simulink model "EHB_MOTOR"  (R2023b)
settings: Solver=FixedStepDiscrete  StartTime=0.0  StopTime=inf  FixedStep=0.0001  RelTol=1e-3  EnableMultiTasking=on
undefined symbols (not defined in the file): CAN_EHB_VCU0x125, CAN_EHB_VCU0x126, CAN_id0x120_Data, Cos_Table, Cos_Table1, EHB_DTC_status, R, Sin_BreakPoint, Sin_BreakPoint1, Sin_Table, Sin_Table1, T
libraries: simulink x30
(part 5 of 9)

== system EHB_MOTOR/EHB_MOTOR_PRO/DIAG/EHBDiag/Subsystem ==
  note: 电源电压过高
  note: 11V
  note: 16V
  note: 电源电压过低
  note: 9V
  note: 14V
  In1 : Inport
  function : TriggerPort  TriggerType=function-call  VariantControl=Variant
  Constant{,1..3} (4 alike) : Constant  Value=0  OutDataTypeStr=uint8
  Data Store Memory1 : DataStoreMemory  DataStoreName=EHBVoltage_C  ReadBeforeWriteMsg=warning  WriteAfterWriteMsg=warning  WriteAfterReadMsg=warning  ShowAdditionalParam=off  OutDataTypeStr=uint16
  Data Store Memory2 : DataStoreMemory  DataStoreName=EHBVoltageMIN2_C  ReadBeforeWriteMsg=warning  WriteAfterWriteMsg=warning  WriteAfterReadMsg=warning  ShowAdditionalParam=off  OutDataTypeStr=uint16
  Data Store Memory3 : DataStoreMemory  DataStoreName=EHBVoltageMAX2_C  ReadBeforeWriteMsg=warning  WriteAfterWriteMsg=warning  WriteAfterReadMsg=warning  ShowAdditionalParam=off  OutDataTypeStr=uint16
  Data Store Memory4 : DataStoreMemory  DataStoreName=EHBVoltageMIN1_C  ReadBeforeWriteMsg=warning  WriteAfterWriteMsg=warning  WriteAfterReadMsg=warning  ShowAdditionalParam=off  OutDataTypeStr=uint16
  Data Store Memory5 : DataStoreMemory  DataStoreName=EHBVoltageMAX1_C  ReadBeforeWriteMsg=warning  WriteAfterWriteMsg=warning  WriteAfterReadMsg=warning  ShowAdditionalParam=off  OutDataTypeStr=uint16
  Data Store Read : DataStoreRead  DataStoreName=EHBVoltage_C  DataStoreElements=EHBVoltage_C  IndexOptions=Index vector (dialog)  Indices=1  OutputSizes=1
  Data Store Read1 : DataStoreRead  DataStoreName=EHBVoltageMIN1_C  DataStoreElements=EHBVoltageMIN1_C  IndexOptions=Index vector (dialog)  Indices=1  OutputSizes=1
  Data Store Read2 : DataStoreRead  DataStoreName=EHBVoltageMAX1_C  DataStoreElements=EHBVoltageMAX1_C  IndexOptions=Index vector (dialog)  Indices=1  OutputSizes=1
  Data Store Read3 : DataStoreRead  DataStoreName=EHBVoltageMAX2_C  DataStoreElements=EHBVoltageMAX2_C  IndexOptions=Index vector (dialog)  Indices=1  OutputSizes=1
  Data Store Read5 : DataStoreRead  DataStoreName=EHBVoltageMIN2_C  DataStoreElements=EHBVoltageMIN2_C  IndexOptions=Index vector (dialog)  Indices=1  OutputSizes=1
  ErrorSignalCount : Stateflow chart  TreatAsAtomicUnit=on
  ErrorSignalCount1 : Stateflow chart  TreatAsAtomicUnit=on
  ErrorSignalCount2 : Stateflow chart  TreatAsAtomicUnit=on
  ErrorSignalCount3 : Stateflow chart  TreatAsAtomicUnit=on
  Relational Operator : RelationalOperator  Operator=<  OutDataTypeStr=boolean  RndMeth=Simplest  InputSameDT=off
  Relational Operator1 : RelationalOperator  Operator=>  OutDataTypeStr=boolean  RndMeth=Simplest  InputSameDT=off
  Relational Operator2 : RelationalOperator  Operator=<  OutDataTypeStr=boolean  RndMeth=Simplest  InputSameDT=off
  Relational Operator3 : RelationalOperator  Operator=>  OutDataTypeStr=boolean  RndMeth=Simplest  InputSameDT=off
  EHBVoltageLow1 : Outport  VectorParamsAs1DForOutWhenUnconnected=off
  EHBVoltageLow2 : Outport  Port=2  VectorParamsAs1DForOutWhenUnconnected=off
  EHBVoltageHigh1 : Outport  Port=3  VectorParamsAs1DForOutWhenUnconnected=off
  EHBVoltageHigh2 : Outport  Port=4  VectorParamsAs1DForOutWhenUnconnected=off
  wires:
  Data Store Read1/1 -> Relational Operator/2
  In1/1 -> Relational Operator/1, Relational Operator2/1, Relational Operator1/1, Relational Operator3/1
  Data Store Read2/1 -> Relational Operator1/2
  ErrorSignalCount1/1(EHBVoltageMIN) -> EHBVoltageLow1/1
  Relational Operator/1 -> ErrorSignalCount1/1(EHBVoltage)
  Constant/1 -> ErrorSignalCount1/3(Recover)
  Constant1/1 -> ErrorSignalCount/3(Recover)
  Relational Operator1/1 -> ErrorSignalCount/1(EHBVoltage)
  ErrorSignalCount/1(EHBVoltageMAX) -> EHBVoltageHigh1/1
  Constant2/1 -> ErrorSignalCount2/3(Recover)
  Relational Operator2/1 -> ErrorSignalCount2/1(EHBVoltage)
  Data Store Read5/1 -> Relational Operator2/2
  Data Store Read/1 -> ErrorSignalCount1/2(EHBVoltageMIN_C), ErrorSignalCount2/2(EHBVoltageMIN_C), ErrorSignalCount3/2(EHBVoltageMAX_C), ErrorSignalCount/2(EHBVoltageMAX_C)
  Constant3/1 -> ErrorSignalCount3/3(Recover)
  Data Store Read3/1 -> Relational Operator3/2
  Relational Operator3/1 -> ErrorSignalCount3/1(EHBVoltage)
  ErrorSignalCount2/1(EHBVoltageMIN) -> EHBVoltageLow2/1
  ErrorSignalCount3/1(EHBVoltageMAX) -> EHBVoltageHigh2/1

== system EHB_MOTOR/EHB_MOTOR_PRO/DIAG/KL15VoltageDiag/Subsystem ==
  note: 电源电压过低
  note: 16V
  note: 10V
  note: 电源电压过高
  KL15Voltage : Inport
  function : TriggerPort  TriggerType=function-call  VariantControl=Variant
  Constant : Constant  Value=0  OutDataTypeStr=uint8
  Constant1 : Constant  Value=0  OutDataTypeStr=uint8
  Data Store Memory1 : DataStoreMemory  DataStoreName=KL15Voltage_C  ReadBeforeWriteMsg=warning  WriteAfterWriteMsg=warning  WriteAfterReadMsg=warning  ShowAdditionalParam=off  OutDataTypeStr=uint16
  Data Store Memory4 : DataStoreMemory  DataStoreName=KL15VoltageMIN_C  ReadBeforeWriteMsg=warning  WriteAfterWriteMsg=warning  WriteAfterReadMsg=warning  ShowAdditionalParam=off  OutDataTypeStr=uint16
  Data Store Memory5 : DataStoreMemory  DataStoreName=KL15VoltageMAX_C  ReadBeforeWriteMsg=warning  WriteAfterWriteMsg=warning  WriteAfterReadMsg=warning  ShowAdditionalParam=off  OutDataTypeStr=uint16
  Data Store Read : DataStoreRead  DataStoreName=KL15Voltage_C  DataStoreElements=KL15Voltage_C  IndexOptions=Index vector (dialog)  Indices=1  OutputSizes=1
  Data Store Read1 : DataStoreRead  DataStoreName=KL15VoltageMIN_C  DataStoreElements=KL15VoltageMIN_C  IndexOptions=Index vector (dialog)  Indices=1  OutputSizes=1
  Data Store Read2 : DataStoreRead  DataStoreName=KL15VoltageMAX_C  DataStoreElements=KL15VoltageMAX_C  IndexOptions=Index vector (dialog)  Indices=1  OutputSizes=1
  Data Store Read3 : DataStoreRead  DataStoreName=KL15Voltage_C  DataStoreElements=KL15Voltage_C  IndexOptions=Index vector (dialog)  Indices=1  OutputSizes=1
  ErrorSignalCount : Stateflow chart  TreatAsAtomicUnit=on
  ErrorSignalCount1 : Stateflow chart  TreatAsAtomicUnit=on
  Relational Operator : RelationalOperator  Operator=<  OutDataTypeStr=boolean  RndMeth=Simplest  InputSameDT=off
  Relational Operator1 : RelationalOperator  Operator=>  OutDataTypeStr=boolean  RndMeth=Simplest  InputSameDT=off
  KL15VoltageLow : Outport  VectorParamsAs1DForOutWhenUnconnected=off
  KL15VoltageHigh : Outport  Port=2  VectorParamsAs1DForOutWhenUnconnected=off
  wires:
  ErrorSignalCount/1(KL15VoltageMAX) -> KL15VoltageHigh/1
  Relational Operator1/1 -> ErrorSignalCount/1(KL15Voltage)
  Data Store Read3/1 -> ErrorSignalCount/2(KL15VoltageMAX_C)
  Constant1/1 -> ErrorSignalCount/3(Recover)
  Constant/1 -> ErrorSignalCount1/3(Recover)
  Data Store Read/1 -> ErrorSignalCount1/2(KL15VoltageMIN_C)
  Relational Operator/1 -> ErrorSignalCount1/1(KL15Voltage)
  ErrorSignalCount1/1(KL15VoltageMIN) -> KL15VoltageLow/1
  Data Store Read2/1 -> Relational Operator1/2
  KL15Voltage/1 -> Relational Operator/1, Relational Operator1/1
  Data Store Read1/1 -> Relational Operator/2

== system EHB_MOTOR/EHB_MOTOR_PRO/DIAG/LogicVoltageDiag/Subsystem ==
  note: 电源电压过高
  note: 10V
  note: 16V
  note: 电源电压过低
  In1 : Inport
  function : TriggerPort  TriggerType=function-call  VariantControl=Variant
  Constant : Constant  Value=0  OutDataTypeStr=uint8
  Constant1 : Constant  Value=0  OutDataTypeStr=uint8
  Data Store Memory1 : DataStoreMemory  DataStoreName=LogicVoltage_C  ReadBeforeWriteMsg=warning  WriteAfterWriteMsg=warning  WriteAfterReadMsg=warning  ShowAdditionalParam=off  OutDataTypeStr=uint16
  Data Store Memory4 : DataStoreMemory  DataStoreName=LogicVoltageMIN_C  ReadBeforeWriteMsg=warning  WriteAfterWriteMsg=warning  WriteAfterReadMsg=warning  ShowAdditionalParam=off  OutDataTypeStr=uint16
  Data Store Memory5 : DataStoreMemory  DataStoreName=LogicVoltageMAX_C  ReadBeforeWriteMsg=warning  WriteAfterWriteMsg=warning  WriteAfterReadMsg=warning  ShowAdditionalParam=off  OutDataTypeStr=uint16
  Data Store Read : DataStoreRead  DataStoreName=LogicVoltage_C  DataStoreElements=LogicVoltage_C  IndexOptions=Index vector (dialog)  Indices=1  OutputSizes=1
  Data Store Read1 : DataStoreRead  DataStoreName=LogicVoltageMIN_C  DataStoreElements=LogicVoltageMIN_C  IndexOptions=Index vector (dialog)  Indices=1  OutputSizes=1
  Data Store Read2 : DataStoreRead  DataStoreName=LogicVoltageMAX_C  DataStoreElements=LogicVoltageMAX_C  IndexOptions=Index vector (dialog)  Indices=1  OutputSizes=1
  Data Store Read3 : DataStoreRead  DataStoreName=LogicVoltage_C  DataStoreElements=LogicVoltage_C  IndexOptions=Index vector (dialog)  Indices=1  OutputSizes=1
  ErrorSignalCount : Stateflow chart  TreatAsAtomicUnit=on
  ErrorSignalCount1 : Stateflow chart  TreatAsAtomicUnit=on
  Relational Operator : RelationalOperator  Operator=<  OutDataTypeStr=boolean  RndMeth=Simplest  InputSameDT=off
  Relational Operator1 : RelationalOperator  Operator=>  OutDataTypeStr=boolean  RndMeth=Simplest  InputSameDT=off
  Out1 : Outport  VectorParamsAs1DForOutWhenUnconnected=off
  Out2 : Outport  Port=2  VectorParamsAs1DForOutWhenUnconnected=off
  wires:
  Data Store Read1/1 -> Relational Operator/2
  In1/1 -> Relational Operator/1, Relational Operator1/1
  Data Store Read2/1 -> Relational Operator1/2
  ErrorSignalCount1/1(LogicVoltageMIN) -> Out1/1
  Relational Operator/1 -> ErrorSignalCount1/1(LogicVoltage)
  Data Store Read/1 -> ErrorSignalCount1/2(LogicVoltageMIN_C)
  Constant/1 -> ErrorSignalCount1/3(Recover)
  Constant1/1 -> ErrorSignalCount/3(Recover)
  Data Store Read3/1 -> ErrorSignalCount/2(LogicVoltageMAX_C)
  Relational Operator1/1 -> ErrorSignalCount/1(LogicVoltage)
  ErrorSignalCount/1(LogicVoltageMAX) -> Out2/1

== system EHB_MOTOR/EHB_MOTOR_PRO/DIAG/MotorDiag/Subsystem ==
  note: 电机回路开路或短路
  In1 : Inport
  Motor_PWMout : Inport  Port=2
  function : TriggerPort  TriggerType=function-call  VariantControl=Variant
  Abs : Abs  SaturateOnIntegerOverflow=off
  Constant : Constant  Value=0
  Constant1 : Constant  Value=500
  Constant2 : Constant  Value=500
  Data Store Memory1 : DataStoreMemory  DataStoreName=MotorCircuitCurrentOverride_C  ReadBeforeWriteMsg=warning  WriteAfterWriteMsg=warning  WriteAfterReadMsg=warning  ShowAdditionalParam=off  OutDataTypeStr=uint8
  Data Store Memory4 : DataStoreMemory  DataStoreName=MotorCircuitCurrentMIN_C  ReadBeforeWriteMsg=warning  WriteAfterWriteMsg=warning  WriteAfterReadMsg=warning  ShowAdditionalParam=off  OutDataTypeStr=uint16
  Data Store Memory5 : DataStoreMemory  DataStoreName=MotorCircuitCurrentMAX_C  ReadBeforeWriteMsg=warning  WriteAfterWriteMsg=warning  WriteAfterReadMsg=warning  ShowAdditionalParam=off  OutDataTypeStr=uint16
  Data Store Read : DataStoreRead  DataStoreName=MotorCircuitCurrentOverride_C  DataStoreElements=MotorCircuitCurrentOverride_C  IndexOptions=Index vector (dialog)  Indices=1  OutputSizes=1
  Data Store Read1 : DataStoreRead  DataStoreName=MotorCircuitCurrentMIN_C  DataStoreElements=MotorCircuitCurrentMIN_C  IndexOptions=Index vector (dialog)  Indices=1  OutputSizes=1
  Data Store Read2 : DataStoreRead  DataStoreName=MotorCircuitCurrentMAX_C  DataStoreElements=MotorCircuitCurrentMAX_C  IndexOptions=Index vector (dialog)  Indices=1  OutputSizes=1
  ErrorSignalCount : Stateflow chart  TreatAsAtomicUnit=on
  Logical Operator : Logic  Operator=OR  AllPortsSameDT=off  OutDataTypeStr=boolean
  Logical Operator1 : Logic  AllPortsSameDT=off  OutDataTypeStr=boolean
  Logical Operator2 : Logic  AllPortsSameDT=off  OutDataTypeStr=boolean
  Relational Operator : RelationalOperator  Operator=<  OutDataTypeStr=boolean  RndMeth=Simplest  InputSameDT=off
  Relational Operator1 : RelationalOperator  Operator=>  OutDataTypeStr=boolean  RndMeth=Simplest  InputSameDT=off
  Relational Operator2 : RelationalOperator  Operator===  OutDataTypeStr=boolean  RndMeth=Simplest  InputSameDT=off
  Relational Operator3 : RelationalOperator  Operator=~=  OutDataTypeStr=boolean  RndMeth=Simplest  InputSameDT=off
  Out1 : Outport  VectorParamsAs1DForOutWhenUnconnected=off
  wires:
  Constant/1 -> ErrorSignalCount/3(Recover)
  Data Store Read/1 -> ErrorSignalCount/2(MotorCircuitCurrentOverride_C)
  Logical Operator/1 -> ErrorSignalCount/1(MotorCircuitCurrent)
  ErrorSignalCount/1(MotorCircuitCurrentOverride) -> Out1/1
  Data Store Read2/1 -> Relational Operator1/2
  In1/1 -> Abs/1
  Data Store Read1/1 -> Relational Operator/2
  Abs/1 -> Relational Operator/1, Relational Operator1/1
  Constant1/1 -> Relational Operator2/2
  Relational Operator1/1 -> Logical Operator1/1
  Relational Operator2/1 -> Logical Operator1/2
  Logical Operator1/1 -> Logical Operator/2
  Relational Operator3/1 -> Logical Operator2/1
  Motor_PWMout/1 -> Relational Operator3/1, Relational Operator2/1
  Constant2/1 -> Relational Operator3/2
  Relational Operator/1 -> Logical Operator2/2
  Logical Operator2/1 -> Logical Operator/1

== system EHB_MOTOR/EHB_MOTOR_PRO/DIAG/MotorDiag/Subsystem1 ==
  note: 电机内部故障或堵转
  In1 : Inport
  function : TriggerPort  TriggerType=function-call  VariantControl=Variant
  Constant : Constant  Value=0
  Data Store Memory1 : DataStoreMemory  DataStoreName=MotorTempOverride_C  ReadBeforeWriteMsg=warning  WriteAfterWriteMsg=warning  WriteAfterReadMsg=warning  ShowAdditionalParam=off  OutDataTypeStr=uint8
  Data Store Memory5 : DataStoreMemory  DataStoreName=MotorTempMAX_C  ReadBeforeWriteMsg=warning  WriteAfterWriteMsg=warning  WriteAfterReadMsg=warning  ShowAdditionalParam=off  OutDataTypeStr=uint16
  Data Store Read : DataStoreRead  DataStoreName=MotorTempOverride_C  DataStoreElements=MotorTempOverride_C  IndexOptions=Index vector (dialog)  Indices=1  OutputSizes=1
  Data Store Read2 : DataStoreRead  DataStoreName=MotorTempMAX_C  DataStoreElements=MotorTempMAX_C  IndexOptions=Index vector (dialog)  Indices=1  OutputSizes=1
  ErrorSignalCount : Stateflow chart  TreatAsAtomicUnit=on
  Relational Operator1 : RelationalOperator  Operator=>  OutDataTypeStr=boolean  RndMeth=Simplest  InputSameDT=off
  Out1 : Outport  VectorParamsAs1DForOutWhenUnconnected=off
  wires:
  ErrorSignalCount/1(MotorTempOverride) -> Out1/1
  Relational Operator1/1 -> ErrorSignalCount/1(MotorTemp)
  Data Store Read/1 -> ErrorSignalCount/2(MotorTempOverride_C)
  Constant/1 -> ErrorSignalCount/3(Recover)
  In1/1 -> Relational Operator1/1
  Data Store Read2/1 -> Relational Operator1/2

== system EHB_MOTOR/EHB_MOTOR_PRO/DIAG/MotorDiag/Subsystem2 ==
  note: 电机内部故障或堵转
  In1 : Inport
  function : TriggerPort  TriggerType=function-call  VariantControl=Variant
  Abs : Abs  SaturateOnIntegerOverflow=off
  Constant : Constant  Value=0
  Data Store Memory1 : DataStoreMemory  DataStoreName=MotorCurrentOverride_C  ReadBeforeWriteMsg=warning  WriteAfterWriteMsg=warning  WriteAfterReadMsg=warning  ShowAdditionalParam=off  OutDataTypeStr=uint8
  Data Store Memory5 : DataStoreMemory  DataStoreName=MotorCurrentMAX_C  ReadBeforeWriteMsg=warning  WriteAfterWriteMsg=warning  WriteAfterReadMsg=warning  ShowAdditionalParam=off  OutDataTypeStr=uint16
  Data Store Read : DataStoreRead  DataStoreName=MotorCurrentOverride_C  DataStoreElements=MotorCurrentOverride_C  IndexOptions=Index vector (dialog)  Indices=1  OutputSizes=1
  Data Store Read2 : DataStoreRead  DataStoreName=MotorCurrentMAX_C  DataStoreElements=MotorCurrentMAX_C  IndexOptions=Index vector (dialog)  Indices=1  OutputSizes=1
  ErrorSignalCount : Stateflow chart  TreatAsAtomicUnit=on
  Relational Operator1 : RelationalOperator  Operator=>  OutDataTypeStr=boolean  RndMeth=Simplest  InputSameDT=off
  Out1 : Outport  VectorParamsAs1DForOutWhenUnconnected=off
  wires:
  In1/1 -> Abs/1
  Data Store Read2/1 -> Relational Operator1/2
  ErrorSignalCount/1(MotorCurrentOverride) -> Out1/1
  Relational Operator1/1 -> ErrorSignalCount/1(MotorCurrent)
  Data Store Read/1 -> ErrorSignalCount/2(MotorCurrentOverride_C)
  Constant/1 -> ErrorSignalCount/3(Recover)
  Abs/1 -> Relational Operator1/1

== system EHB_MOTOR/EHB_MOTOR_PRO/DIAG/PressureSensorDiag/Subsystem ==
  note: 压力信号超过限定值
  VCU_Brake_AimPressure : Inport
  EHB_actPresure_filtered : Inport  Port=2
  function : TriggerPort  TriggerType=function-call  VariantControl=Variant
  Abs : Abs  SaturateOnIntegerOverflow=off
  Add : Sum  Inputs=+-
  Constant : Constant  Value=0  OutDataTypeStr=uint8
  Constant1 : Constant  Value=0  OutDataTypeStr=uint8
  Data Store Memory1 : DataStoreMemory  DataStoreName=PressureSensorSignalOverride_C  ReadBeforeWriteMsg=warning  WriteAfterWriteMsg=warning  WriteAfterReadMsg=warning  ShowAdditionalParam=off  OutDataTypeStr=uint16
  Data Store Memory4 : DataStoreMemory  DataStoreName=PressureSensorSignalMIN_C  ReadBeforeWriteMsg=warning  WriteAfterWriteMsg=warning  WriteAfterReadMsg=warning  ShowAdditionalParam=off  OutDataTypeStr=uint16
  Data Store Memory5 : DataStoreMemory  DataStoreName=PressureSensorSignalMAX_C  ReadBeforeWriteMsg=warning  WriteAfterWriteMsg=warning  WriteAfterReadMsg=warning  ShowAdditionalParam=off  OutDataTypeStr=uint16
  Data Store Read : DataStoreRead  DataStoreName=PressureSensorSignalOverride_C  DataStoreElements=PressureSensorSignalOverride_C  IndexOptions=Index vector (dialog)  Indices=1  OutputSizes=1
  Data Store Read1 : DataStoreRead  DataStoreName=PressureSensorSignalMIN_C  DataStoreElements=PressureSensorSignalMIN_C  IndexOptions=Index vector (dialog)  Indices=1  OutputSizes=1
  Data Store Read2 : DataStoreRead  DataStoreName=PressureSensorSignalMAX_C  DataStoreElements=PressureSensorSignalMAX_C  IndexOptions=Index vector (dialog)  Indices=1  OutputSizes=1
  ErrorSignalCount : Stateflow chart  TreatAsAtomicUnit=on
  ErrorSignalCount1 : Stateflow chart  TreatAsAtomicUnit=on
  Relational Operator : RelationalOperator  Operator=>  OutDataTypeStr=boolean  RndMeth=Simplest  InputSameDT=off
  Relational Operator1 : RelationalOperator  Operator=>  OutDataTypeStr=boolean  RndMeth=Simplest  InputSameDT=off
  Out1 : Outport  VectorParamsAs1DForOutWhenUnconnected=off
  Out2 : Outport  Port=2  VectorParamsAs1DForOutWhenUnconnected=off
  wires:
  Constant/1 -> ErrorSignalCount/3(Recover)
  Data Store Read/1 -> ErrorSignalCount/2(PressureSensorSignalOverride_C), ErrorSignalCount1/2(PressureSensorSignalOverride_C)
  Relational Operator/1 -> ErrorSignalCount/1(PressureSensorSignal)
  Relational Operator1/1 -> ErrorSignalCount1/1(PressureSensorSignal)
  ErrorSignalCount/1(PressureSensorSignalOverride) -> Out1/1
  Data Store Read2/1 -> Relational Operator1/2
  Data Store Read1/1 -> Relational Operator/2
  VCU_Brake_AimPressure/1 -> Add/1
  EHB_actPresure_filtered/1 -> Add/2
  Add/1 -> Abs/1
  Abs/1 -> Relational Operator/1, Relational Operator1/1
  Constant1/1 -> ErrorSignalCount1/3(Recover)
  ErrorSignalCount1/1(PressureSensorSignalOverride) -> Out2/1

== system EHB_MOTOR/EHB_MOTOR_PRO/DIAG/PressureSensorDiag/Subsystem1 ==
  note: 压力传感器信号在一定时间内没有反馈
  EHB_Presure_ADC : Inport
  function : TriggerPort  TriggerType=function-call  VariantControl=Variant
  Constant : Constant  Value=0  OutDataTypeStr=uint8
  Constant1 : Constant  Value=300
  Constant2 : Constant  Value=2550
  Data Store Memory1 : DataStoreMemory  DataStoreName=PressureSensorSignalLost_C  ReadBeforeWriteMsg=warning  WriteAfterWriteMsg=warning  WriteAfterReadMsg=warning  ShowAdditionalParam=off  OutDataTypeStr=uint16
  Data Store Read : DataStoreRead  DataStoreName=PressureSensorSignalLost_C  DataStoreElements=PressureSensorSignalLost_C  IndexOptions=Index vector (dialog)  Indices=1  OutputSizes=1
  ErrorSignalCount : Stateflow chart  TreatAsAtomicUnit=on
  Logical Operator : Logic  Operator=OR  AllPortsSameDT=off  OutDataTypeStr=boolean
  Relational Operator : RelationalOperator  Operator=<  OutDataTypeStr=boolean  RndMeth=Simplest  InputSameDT=off
  Relational Operator1 : RelationalOperator  Operator=>  OutDataTypeStr=boolean  RndMeth=Simplest  InputSameDT=off
  Out1 : Outport  VectorParamsAs1DForOutWhenUnconnected=off
  wires:
  Constant1/1 -> Relational Operator/2
  EHB_Presure_ADC/1 -> Relational Operator/1, Relational Operator1/1
  ErrorSignalCount/1(PressureSensorSignalLost) -> Out1/1
  Data Store Read/1 -> ErrorSignalCount/2(PressureSensorSignalLost_C)
  Constant/1 -> ErrorSignalCount/3(Recover)
  Constant2/1 -> Relational Operator1/2
  Relational Operator1/1 -> Logical Operator/1
  Relational Operator/1 -> Logical Operator/2
  Logical Operator/1 -> ErrorSignalCount/1(PressureSensorSignal)

== system EHB_MOTOR/EHB_MOTOR_PRO/DIAG/PressureSensorDiag/Subsystem2 ==
  note: 压力传感器标定状态位为0
  In1 : Inport
  function : TriggerPort  TriggerType=function-call  VariantControl=Variant
  Constant : Constant  Value=0  OutDataTypeStr=uint8
  Constant1 : Constant  Value=0
  Data Store Memory1 : DataStoreMemory  DataStoreName=PressureSensorNoCal_C  ReadBeforeWriteMsg=warning  WriteAfterWriteMsg=warning  WriteAfterReadMsg=warning  ShowAdditionalParam=off  OutDataTypeStr=uint16
  Data Store Read : DataStoreRead  DataStoreName=PressureSensorNoCal_C  DataStoreElements=PressureSensorNoCal_C  IndexOptions=Index vector (dialog)  Indices=1  OutputSizes=1
  ErrorSignalCount : Stateflow chart  TreatAsAtomicUnit=on
  Relational Operator : RelationalOperator  Operator===  OutDataTypeStr=boolean  RndMeth=Simplest  InputSameDT=off
  Out1 : Outport  VectorParamsAs1DForOutWhenUnconnected=off
  wires:
  Constant/1 -> ErrorSignalCount/3(Recover)
  Data Store Read/1 -> ErrorSignalCount/2(PressureSensorNoCal_C)
  Relational Operator/1 -> ErrorSignalCount/1(PressureSensorSignal)
  ErrorSignalCount/1(PressureSensorNoCal) -> Out1/1
  In1/1 -> Relational Operator/1
  Constant1/1 -> Relational Operator/2

== system EHB_MOTOR/EHB_MOTOR_PRO/DIAG/SpeedSensorDiag/Subsystem ==
  note: 监测到轮速传感器电压信号电压超出范围[0.2,1]
  note: 0.2
  note: 1
  In1 : Inport
  function : TriggerPort  TriggerType=function-call  VariantControl=Variant
  Constant : Constant  Value=0  OutDataTypeStr=uint8
  Data Store Memory1 : DataStoreMemory  DataStoreName=SpeedSensorOverride_C  ReadBeforeWriteMsg=warning  WriteAfterWriteMsg=warning  WriteAfterReadMsg=warning  ShowAdditionalParam=off  OutDataTypeStr=uint16
  Data Store Memory4 : DataStoreMemory  DataStoreName=SpeedSensorMIN_C  ReadBeforeWriteMsg=warning  WriteAfterWriteMsg=warning  WriteAfterReadMsg=warning  ShowAdditionalParam=off  OutDataTypeStr=uint16
  Data Store Memory5 : DataStoreMemory  DataStoreName=SpeedSensorMAX_C  ReadBeforeWriteMsg=warning  WriteAfterWriteMsg=warning  WriteAfterReadMsg=warning  ShowAdditionalParam=off  OutDataTypeStr=uint16
  Data Store Read : DataStoreRead  DataStoreName=SpeedSensorOverride_C  DataStoreElements=SpeedSensorOverride_C  IndexOptions=Index vector (dialog)  Indices=1  OutputSizes=1
  Data Store Read1 : DataStoreRead  DataStoreName=SpeedSensorMIN_C  DataStoreElements=SpeedSensorMIN_C  IndexOptions=Index vector (dialog)  Indices=1  OutputSizes=1
  Data Store Read2 : DataStoreRead  DataStoreName=SpeedSensorMAX_C  DataStoreElements=SpeedSensorMAX_C  IndexOptions=Index vector (dialog)  Indices=1  OutputSizes=1
  ErrorSignalCount : Stateflow chart  TreatAsAtomicUnit=on
  Logical Operator : Logic  Operator=OR  AllPortsSameDT=off  OutDataTypeStr=boolean
  Relational Operator : RelationalOperator  Operator=<  OutDataTypeStr=boolean  RndMeth=Simplest  InputSameDT=off
  Relational Operator1 : RelationalOperator  Operator=>  OutDataTypeStr=boolean  RndMeth=Simplest  InputSameDT=off
  Out1 : Outport  VectorParamsAs1DForOutWhenUnconnected=off
  wires:
  Data Store Read1/1 -> Relational Operator/2
  In1/1 -> Relational Operator/1, Relational Operator1/1
  Data Store Read2/1 -> Relational Operator1/2
  ErrorSignalCount/1(SpeedSensorOverride) -> Out1/1
  Relational Operator1/1 -> Logical Operator/2
  Relational Operator/1 -> Logical Operator/1
  Logical Operator/1 -> ErrorSignalCount/1(SpeedSensor)
  Data Store Read/1 -> ErrorSignalCount/2(SpeedSensorOverride_C)
  Constant/1 -> ErrorSignalCount/3(Recover)

== system EHB_MOTOR/EHB_MOTOR_PRO/DIAG/TempDiag/Subsystem1 ==
  note: 温度反馈信号超过限定值
  In1 : Inport
  function : TriggerPort  TriggerType=function-call  VariantControl=Variant
  Constant : Constant  Value=0  OutDataTypeStr=uint8
  Data Store Memory1 : DataStoreMemory  DataStoreName=TempSensorOverride_C  ReadBeforeWriteMsg=warning  WriteAfterWriteMsg=warning  WriteAfterReadMsg=warning  ShowAdditionalParam=off  OutDataTypeStr=uint16
  Data Store Memory5 : DataStoreMemory  DataStoreName=TempSensorMAX_C  ReadBeforeWriteMsg=warning  WriteAfterWriteMsg=warning  WriteAfterReadMsg=warning  ShowAdditionalParam=off  OutDataTypeStr=uint16
  Data Store Read : DataStoreRead  DataStoreName=TempSensorOverride_C  DataStoreElements=TempSensorOverride_C  IndexOptions=Index vector (dialog)  Indices=1  OutputSizes=1
  Data Store Read2 : DataStoreRead  DataStoreName=TempSensorMAX_C  DataStoreElements=TempSensorMAX_C  IndexOptions=Index vector (dialog)  Indices=1  OutputSizes=1
  ErrorSignalCount : Stateflow chart  TreatAsAtomicUnit=on
  Relational Operator1 : RelationalOperator  Operator=>  OutDataTypeStr=boolean  RndMeth=Simplest  InputSameDT=off
  Out1 : Outport  VectorParamsAs1DForOutWhenUnconnected=off
  wires:
  ErrorSignalCount/1(TempSensorOverride) -> Out1/1
  Relational Operator1/1 -> ErrorSignalCount/1(TempSensor)
  Data Store Read/1 -> ErrorSignalCount/2(TempSensorOverride_C)
  Constant/1 -> ErrorSignalCount/3(Recover)
  Data Store Read2/1 -> Relational Operator1/2
  In1/1 -> Relational Operator1/1

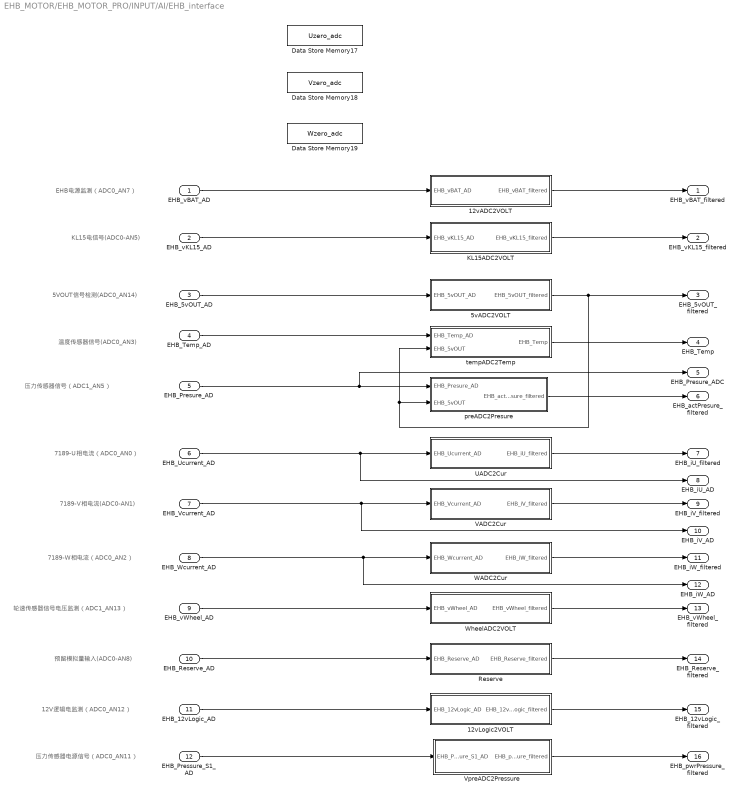
== system EHB_MOTOR/EHB_MOTOR_PRO/INPUT/AI/EHB_interface ==
  note: 12V逻辑电监测（ADC0_AN12）
  note: 预留模拟量输入(ADC0-AN8)
  note: 轮速传感器信号电压监测（ADC1_AN13）
  note: EHB电源监测（ADC0_AN7）
  note: 5VOUT信号检测(ADC0_AN14)
  note: KL15电信号(ADC0-AN5)
  note: 温度传感器信号(ADC0_AN3)
  note: 压力传感器信号（ADC1_AN5）
  note: 7189-W相电流（ADC0_AN2）
  note: 7189-U相电流（ADC0_AN0）
  note: 7189-V相电流(ADC0-AN1)
  note: 压力传感器电源信号（ADC0_AN11）
  EHB_vBAT_AD : Inport
  EHB_vKL15_AD : Inport  Port=2
  EHB_5vOUT_AD : Inport  Port=3
  EHB_Temp_AD : Inport  Port=4
  EHB_Presure_AD : Inport  Port=5
  EHB_Ucurrent_AD : Inport  Port=6
  EHB_Vcurrent_AD : Inport  Port=7
  EHB_Wcurrent_AD : Inport  Port=8
  EHB_vWheel_AD : Inport  Port=9
  EHB_Reserve_AD : Inport  Port=10
  EHB_12vLogic_AD : Inport  Port=11
  EHB_Pressure_S1_AD : Inport  Port=12
  12vADC2VOLT : Subsystem
  12vLogic2VOLT : Subsystem
  5vADC2VOLT : Subsystem
  Data Store Memory17 : DataStoreMemory  DataStoreName=Uzero_adc  ReadBeforeWriteMsg=warning  WriteAfterWriteMsg=warning  WriteAfterReadMsg=warning  ShowAdditionalParam=off  OutDataTypeStr=uint16
  Data Store Memory18 : DataStoreMemory  DataStoreName=Vzero_adc  ReadBeforeWriteMsg=warning  WriteAfterWriteMsg=warning  WriteAfterReadMsg=warning  ShowAdditionalParam=off  OutDataTypeStr=uint16
  Data Store Memory19 : DataStoreMemory  DataStoreName=Wzero_adc  ReadBeforeWriteMsg=warning  WriteAfterWriteMsg=warning  WriteAfterReadMsg=warning  ShowAdditionalParam=off  OutDataTypeStr=uint16
  KL15ADC2VOLT : Subsystem
  Reserve : Subsystem
  UADC2Cur : Subsystem
  VADC2Cur : Subsystem
  VpreADC2Pressure : Subsystem
  WADC2Cur : Subsystem
  WheelADC2VOLT : Subsystem
  preADC2Presure : Subsystem
  tempADC2Temp : Subsystem
  EHB_vBAT_filtered : Outport  VectorParamsAs1DForOutWhenUnconnected=off
  EHB_vKL15_filtered : Outport  Port=2  VectorParamsAs1DForOutWhenUnconnected=off
  EHB_5vOUT_filtered : Outport  Port=3  VectorParamsAs1DForOutWhenUnconnected=off
  EHB_Temp : Outport  Port=4  VectorParamsAs1DForOutWhenUnconnected=off
  EHB_Presure_ADC : Outport  Port=5  VectorParamsAs1DForOutWhenUnconnected=off
  EHB_actPresure_filtered : Outport  Port=6  VectorParamsAs1DForOutWhenUnconnected=off
  EHB_iU_filtered : Outport  Port=7  VectorParamsAs1DForOutWhenUnconnected=off
  EHB_iU_AD : Outport  Port=8  VectorParamsAs1DForOutWhenUnconnected=off
  EHB_iV_filtered : Outport  Port=9  VectorParamsAs1DForOutWhenUnconnected=off
  EHB_iV_AD : Outport  Port=10  VectorParamsAs1DForOutWhenUnconnected=off
  EHB_iW_filtered : Outport  Port=11  VectorParamsAs1DForOutWhenUnconnected=off
  EHB_iW_AD : Outport  Port=12  VectorParamsAs1DForOutWhenUnconnected=off
  EHB_vWheel_filtered : Outport  Port=13  VectorParamsAs1DForOutWhenUnconnected=off
  EHB_Reserve_filtered : Outport  Port=14  VectorParamsAs1DForOutWhenUnconnected=off
  EHB_12vLogic_filtered : Outport  Port=15  VectorParamsAs1DForOutWhenUnconnected=off
  EHB_pwrPressure_filtered : Outport  Port=16  VectorParamsAs1DForOutWhenUnconnected=off
  wires:
  12vADC2VOLT/1(EHB_vBAT_filtered) -> EHB_vBAT_filtered/1
  KL15ADC2VOLT/1(EHB_vKL15_filtered) -> EHB_vKL15_filtered/1
  5vADC2VOLT/1(EHB_5vOUT_filtered) -> EHB_5vOUT_filtered/1, tempADC2Temp/2(EHB_5vOUT), preADC2Presure/2(EHB_5vOUT)
  preADC2Presure/1(EHB_actPresure_filtered) -> EHB_actPresure_filtered/1
  UADC2Cur/1(EHB_iU_filtered) -> EHB_iU_filtered/1
  VADC2Cur/1(EHB_iV_filtered) -> EHB_iV_filtered/1
  WADC2Cur/1(EHB_iW_filtered) -> EHB_iW_filtered/1
  WheelADC2VOLT/1(EHB_vWheel_filtered) -> EHB_vWheel_filtered/1
  EHB_vKL15_AD/1 -> KL15ADC2VOLT/1(EHB_vKL15_AD)
  EHB_Temp_AD/1 -> tempADC2Temp/1(EHB_Temp_AD)
  EHB_5vOUT_AD/1 -> 5vADC2VOLT/1(EHB_5vOUT_AD)
  EHB_Presure_AD/1 -> preADC2Presure/1(EHB_Presure_AD), EHB_Presure_ADC/1
  EHB_vBAT_AD/1 -> 12vADC2VOLT/1(EHB_vBAT_AD)
  EHB_Vcurrent_AD/1 -> VADC2Cur/1(EHB_Vcurrent_AD), EHB_iV_AD/1
  EHB_Ucurrent_AD/1 -> UADC2Cur/1(EHB_Ucurrent_AD), EHB_iU_AD/1
  EHB_vWheel_AD/1 -> WheelADC2VOLT/1(EHB_vWheel_AD)
  EHB_Wcurrent_AD/1 -> WADC2Cur/1(EHB_Wcurrent_AD), EHB_iW_AD/1
  EHB_Reserve_AD/1 -> Reserve/1(EHB_Reserve_AD)
  Reserve/1(EHB_Reserve_filtered) -> EHB_Reserve_filtered/1
  EHB_12vLogic_AD/1 -> 12vLogic2VOLT/1(EHB_12vLogic_AD)
  12vLogic2VOLT/1(EHB_12vLogic_filtered) -> EHB_12vLogic_filtered/1
  EHB_Pressure_S1_AD/1 -> VpreADC2Pressure/1(EHB_Pressure_S1_AD)
  VpreADC2Pressure/1(EHB_pwrPressure_filtered) -> EHB_pwrPressure_filtered/1
  tempADC2Temp/1(EHB_Temp) -> EHB_Temp/1

== system EHB_MOTOR/EHB_MOTOR_PRO/OUTPUT/CAN_pack/Subsystem ==
  <EHB_mode> : Inport
  Constant : Constant  Value=2  OutDataTypeStr=Inherit: Inherit via back propagation
  Constant1 : Constant  OutDataTypeStr=uint8
  Constant2 : Constant  Value=0  OutDataTypeStr=uint8
  Relational Operator : RelationalOperator  Operator===  OutDataTypeStr=boolean  RndMeth=Simplest  InputSameDT=off
  Switch : Switch  Criteria=u2 ~= 0  SaturateOnIntegerOverflow=off  InputSameDT=off
  Out1 : Outport  VectorParamsAs1DForOutWhenUnconnected=off
  wires:
  Constant/1 -> Relational Operator/2
  Relational Operator/1 -> Switch/2
  <EHB_mode>/1 -> Relational Operator/1
  Switch/1 -> Out1/1
  Constant2/1 -> Switch/3
  Constant1/1 -> Switch/1

== system EHB_MOTOR/EHB_MOTOR_PRO/OUTPUT/CAN_pack/Subsystem1 ==
  <EHB_mode> : Inport
  Constant : Constant  Value=2  OutDataTypeStr=Inherit: Inherit via back propagation
  Constant1 : Constant  Value=2  OutDataTypeStr=uint8
  Constant2 : Constant  OutDataTypeStr=uint8
  Relational Operator : RelationalOperator  Operator===  OutDataTypeStr=boolean  RndMeth=Simplest  InputSameDT=off
  Switch : Switch  Criteria=u2 ~= 0  SaturateOnIntegerOverflow=off  InputSameDT=off
  Out1 : Outport  VectorParamsAs1DForOutWhenUnconnected=off
  wires:
  Constant1/1 -> Switch/1
  Constant2/1 -> Switch/3
  Switch/1 -> Out1/1
  <EHB_mode>/1 -> Relational Operator/1
  Relational Operator/1 -> Switch/2
  Constant/1 -> Relational Operator/2

== system EHB_MOTOR/EHB_MOTOR_PRO/OUTPUT/CAN_pack/Subsystem2 ==
  In1 : Inport
  Bus Selector : BusSelector  OutputSignals=CurrentSensorUOverride,CurrentSensorVOverride,CurrentSensorWOverride
  Logical Operator : Logic  Operator=OR  Inputs=3  AllPortsSameDT=off  OutDataTypeStr=boolean
  Out1 : Outport  VectorParamsAs1DForOutWhenUnconnected=off
  wires:
  In1/1 -> Bus Selector/1
  Bus Selector/1 -> Logical Operator/1  "<CurrentSensorUOverride>"
  Bus Selector/2 -> Logical Operator/2  "<CurrentSensorVOverride>"
  Bus Selector/3 -> Logical Operator/3  "<CurrentSensorWOverride>"
  Logical Operator/1 -> Out1/1

== system EHB_MOTOR/EHB_MOTOR_PRO/OUTPUT/CAN_pack/Subsystem3 ==
  DIAG_BUS : Inport
  Bus Selector : BusSelector  OutputSignals=EHBVoltageLow1,EHBVoltageHigh1
  Bus Selector1 : BusSelector  OutputSignals=PressureSensorERR,EHBVoltageLow2,EHBVoltageHigh2,CurrentSensorUOverride,CurrentSensorVOverride,CurrentSensorWOverride,TempSensorOverride
  Constant : Constant  Value=4  OutDataTypeStr=uint8
  Constant1 : Constant  OutDataTypeStr=uint8
  Constant2 : Constant  Value=0  OutDataTypeStr=uint8
  Logical Operator : Logic  Operator=OR  AllPortsSameDT=off  OutDataTypeStr=boolean
  Logical Operator1 : Logic  Operator=OR  Inputs=7  AllPortsSameDT=off  OutDataTypeStr=boolean
  Switch : Switch  Criteria=u2 ~= 0  SaturateOnIntegerOverflow=off  InputSameDT=off
  Switch1 : Switch  Criteria=u2 ~= 0  SaturateOnIntegerOverflow=off  InputSameDT=off
  EHB_FltLvl : Outport  VectorParamsAs1DForOutWhenUnconnected=off
  wires:
  DIAG_BUS/1 -> Bus Selector/1, Bus Selector1/1
  Bus Selector/1 -> Logical Operator/1  "<EHBVoltageLow1>"
  Bus Selector/2 -> Logical Operator/2  "<EHBVoltageHigh1>"
  Logical Operator/1 -> Switch/2
  Bus Selector1/1 -> Logical Operator1/1  "<PressureSensorERR>"
  Bus Selector1/2 -> Logical Operator1/2  "<EHBVoltageLow2>"
  Bus Selector1/3 -> Logical Operator1/3  "<EHBVoltageHigh2>"
  Bus Selector1/4 -> Logical Operator1/4  "<CurrentSensorUOverride>"
  Bus Selector1/5 -> Logical Operator1/5  "<CurrentSensorVOverride>"
  Bus Selector1/6 -> Logical Operator1/6  "<CurrentSensorWOverride>"
  Bus Selector1/7 -> Logical Operator1/7  "<TempSensorOverride>"
  Logical Operator1/1 -> Switch1/2
  Constant/1 -> Switch1/1
  Constant1/1 -> Switch/1
  Constant2/1 -> Switch/3
  Switch/1 -> Switch1/3
  Switch1/1 -> EHB_FltLvl/1

== system EHB_MOTOR/EHB_MOTOR_PRO/OUTPUT/FUALT_HANDLE/FLASH_Write ==
  MODE_BUS : Inport
  Bus Selector : BusSelector  OutputSignals=Flash_Ucurrent,Flash_Vcurrent,Flash_Wcurrent
  Data Store Memory1 : DataStoreMemory  DataStoreName=FLASH_iU_ADC  ReadBeforeWriteMsg=warning  WriteAfterWriteMsg=warning  WriteAfterReadMsg=warning  ShowAdditionalParam=off  OutDataTypeStr=uint16
  Data Store Memory2 : DataStoreMemory  DataStoreName=FLASH_iV_ADC  ReadBeforeWriteMsg=warning  WriteAfterWriteMsg=warning  WriteAfterReadMsg=warning  ShowAdditionalParam=off  OutDataTypeStr=uint16
  Data Store Memory3 : DataStoreMemory  DataStoreName=FLASH_iW_ADC  ReadBeforeWriteMsg=warning  WriteAfterWriteMsg=warning  WriteAfterReadMsg=warning  ShowAdditionalParam=off  OutDataTypeStr=uint16
  Data Store Write1 : DataStoreWrite  DataStoreName=FLASH_iU_ADC  DataStoreElements=FLASH_iU_ADC  IndexOptions=Index vector (dialog)  Indices=1  OutputSizes=1
  Data Store Write2 : DataStoreWrite  DataStoreName=FLASH_iV_ADC  DataStoreElements=FLASH_iV_ADC  IndexOptions=Index vector (dialog)  Indices=1  OutputSizes=1
  Data Store Write3 : DataStoreWrite  DataStoreName=FLASH_iW_ADC  DataStoreElements=FLASH_iW_ADC  IndexOptions=Index vector (dialog)  Indices=1  OutputSizes=1
  wires:
  MODE_BUS/1 -> Bus Selector/1
  Bus Selector/1 -> Data Store Write1/1  "<Flash_Ucurrent>"
  Bus Selector/3 -> Data Store Write3/1  "<Flash_Wcurrent>"
  Bus Selector/2 -> Data Store Write2/1  "<Flash_Vcurrent>"

== system EHB_MOTOR/EHB_MOTOR_PRO/OUTPUT/FUALT_HANDLE/Subsystem ==
  In1 : Inport
  Relational Operator : RelationalOperator  Operator=~=  OutDataTypeStr=boolean  RndMeth=Simplest  InputSameDT=off
  Unit Delay : UnitDelay  SampleTime=-1  HasFrameUpgradeWarning=on
  Out1 : Outport  VectorParamsAs1DForOutWhenUnconnected=off
  wires:
  In1/1 -> Relational Operator/1, Unit Delay/1
  Unit Delay/1 -> Relational Operator/2
  Relational Operator/1 -> Out1/1

== system EHB_MOTOR/EHB_MOTOR_PRO/Speed_closed/WeakMagnetism/Subsystem ==
  超前角 : Inport
  n-D Lookup Table : Lookup_n-D  NumberOfTableDimensions=1  BreakpointsForDimension1=Sin_BreakPoint1  BreakpointsForDimension3=[5, 7]  BreakpointsForDimension1DataTypeStr=Inherit: Inherit from 'Breakpoint data'  Table=Sin_Table1  TableDataTypeStr=Inherit: Inherit from 'Table data'  ExtrapMethod=Clip  InternalRulePriority=Speed  OutDataTypeStr=Inherit: Inherit from 'Table data'  RndMeth=Simplest  InputSameDT=off
  n-D Lookup Table1 : Lookup_n-D  NumberOfTableDimensions=1  BreakpointsForDimension1=Sin_BreakPoint1  BreakpointsForDimension3=[5, 7]  BreakpointsForDimension1DataTypeStr=Inherit: Inherit from 'Breakpoint data'  Table=Cos_Table1  TableDataTypeStr=Inherit: Inherit from 'Table data'  ExtrapMethod=Clip  InternalRulePriority=Speed  OutDataTypeStr=Inherit: Inherit from 'Table data'  RndMeth=Simplest  InputSameDT=off
  Sin : Outport  VectorParamsAs1DForOutWhenUnconnected=off
  cos : Outport  Port=2  VectorParamsAs1DForOutWhenUnconnected=off
  wires:
  n-D Lookup Table/1 -> Sin/1
  n-D Lookup Table1/1 -> cos/1
  超前角/1 -> n-D Lookup Table1/1, n-D Lookup Table/1

== system EHB_MOTOR/EHB_MOTOR_PRO/Speed_closed/WeakMagnetism/Subsystem2 ==
  Uerr : Inport
  KP : Inport  Port=2
  Ki : Inport  Port=3
  Add1 : Sum  OutDataTypeStr=single
  Cur_Upper : Constant  Value=0  OutDataTypeStr=single
  Cur_lower : Constant  Value=-1.57  OutDataTypeStr=single
  Delay : Delay  DelayLength=1
  Inte_Sat1 : Saturate  UpperLimit=0  LowerLimit=-1.57
  Inte_Sat2 : Saturate  UpperLimit=0  LowerLimit=-1.57
  Inte_Switch : Switch  SaturateOnIntegerOverflow=off  InputSameDT=off
  Inte_sat_Lower : Switch  Criteria=u2 ~= 0  OutDataTypeStr=single  SaturateOnIntegerOverflow=off  InputSameDT=off
  Inte_sat_Upper : Switch  Criteria=u2 ~= 0  OutDataTypeStr=single  SaturateOnIntegerOverflow=off  InputSameDT=off
  Product3 : Product  OutDataTypeStr=single
  Relational Operator : RelationalOperator  OutDataTypeStr=boolean  RndMeth=Simplest  InputSameDT=off
  Relational Operator1 : RelationalOperator  OutDataTypeStr=boolean  RndMeth=Simplest  InputSameDT=off
  SpeErr_by_I1 : Product  OutDataTypeStr=single
  Sum : Sum  Inputs=|++
  Sum1 : Sum  Inputs=-+|  OutDataTypeStr=single
  Sum3 : Sum  Inputs=|+-  OutDataTypeStr=single
  超前角 : Outport
  wires:
  Inte_Sat1/1 -> 超前角/1
  Uerr/1 -> Product3/1
  Ki/1 -> SpeErr_by_I1/2
  Add1/1 -> Inte_Sat1/1
  KP/1 -> Product3/2
  Inte_sat_Lower/1 -> Inte_Switch/3
  Cur_Upper/1 -> Sum1/2, Relational Operator/2
  Relational Operator/1 -> Inte_sat_Upper/2
  Delay/1 -> Sum/2
  Inte_sat_Upper/1 -> Inte_Switch/1
  Sum3/1 -> Inte_sat_Lower/3
  Product3/1 -> SpeErr_by_I1/1, Add1/1, Sum1/1, Inte_Switch/2, Sum3/2, Relational Operator1/1, Relational Operator/1
  Cur_lower/1 -> Sum3/1, Relational Operator1/2
  Relational Operator1/1 -> Inte_sat_Lower/2
  Sum/1 -> Inte_Sat2/1
  Sum1/1 -> Inte_sat_Upper/1
  SpeErr_by_I1/1 -> Sum/1
  Inte_Switch/1 -> Add1/2, Delay/1
  Inte_Sat2/1 -> Inte_sat_Upper/3, Inte_sat_Lower/1

== system EHB_MOTOR/EHB_MOTOR_PRO/Subsystem/Current_PI/Id_PI ==
  id_desired : Inport
  delta_id : Inport  Port=2  OutDataTypeStr=single
  id_P : Inport  Port=3  OutDataTypeStr=single
  id_I : Inport  Port=4  OutDataTypeStr=single
  u_dc : Inport  Port=5  OutDataTypeStr=single
  Delay : Delay  DelayLength=1
  Gain : Gain  Gain=1.732  OutDataTypeStr=single
  Id_sat : Saturate  UpperLimit=6.65  LowerLimit=-6.65  OutDataTypeStr=single
  Id_sat1 : Saturate  UpperLimit=6.65  LowerLimit=-6.65  OutDataTypeStr=single
  Id_sat2 : Saturate  UpperLimit=6.65  LowerLimit=-6.65  OutDataTypeStr=single
  Product : Product  OutDataTypeStr=single
  Product1 : Product  OutDataTypeStr=single
  Product2 : Product  OutDataTypeStr=single
  Subsystem : Subsystem
  Subsystem1 : Subsystem
  Subsystem2 : Subsystem
  Sum : Sum  OutDataTypeStr=single  InputSameDT=on  SaturateOnIntegerOverflow=on
  Sum1 : Sum  Inputs=|++  OutDataTypeStr=single
  pi_out : Outport  OutDataTypeStr=single  VectorParamsAs1DForOutWhenUnconnected=off
  Ud_out : Outport  Port=2  OutDataTypeStr=single  VectorParamsAs1DForOutWhenUnconnected=off
  wires:
  delta_id/1 -> Product/1  "id_e"
  id_P/1 -> Product/2
  Product/1 -> Subsystem2/2(In2), Product1/1  "yp"
  id_I/1 -> Product1/2
  Id_sat/1 -> pi_out/1
  Sum1/1 -> Id_sat1/1
  Delay/1 -> Subsystem1/2(In2)
  Sum/1 -> Id_sat2/1
  Product2/1 -> Gain/1
  u_dc/1 -> Product2/2
  Gain/1 -> Id_sat/1
  Product1/1 -> Subsystem/2(In2)
  Subsystem/1(Out1) -> Sum1/1
  Subsystem1/1(Out1) -> Sum1/2
  id_desired/1 -> Subsystem2/1(In1), Subsystem1/1(In1), Subsystem/1(In1)
  Subsystem2/1(Out1) -> Sum/1
  Id_sat2/1 -> Ud_out/1, Product2/1
  Id_sat1/1 -> Sum/2, Delay/1

== system EHB_MOTOR/EHB_MOTOR_PRO/Subsystem/Current_PI/Iq_PI ==
  delta_iq : Inport  OutDataTypeStr=single
  iq_p : Inport  Port=2  OutDataTypeStr=single
  iq_I : Inport  Port=3  OutDataTypeStr=single
  U_dc : Inport  Port=4  OutDataTypeStr=single
  Pressure_Cmplt : Inport  Port=5
  VCU_Brake_AimPressure : Inport  Port=6
  EHB_mode : Inport  Port=7
  Constant : Constant  Value=0  OutDataTypeStr=single
  Constant1 : Constant  Value=0  OutDataTypeStr=single
  Constant2 : Constant  Value=0  OutDataTypeStr=single
  Constant3 : Constant  Value=5
  Delay : Delay  DelayLength=1
  Gain : Gain  Gain=1.732  OutDataTypeStr=single
  Iq_sat : Saturate  UpperLimit=6.65  LowerLimit=-6.65  OutDataTypeStr=single
  Iq_sat1 : Saturate  UpperLimit=6.65  LowerLimit=-6.65  OutDataTypeStr=single
  Iq_sat2 : Saturate  UpperLimit=6.65  LowerLimit=-6.65  OutDataTypeStr=single
  Logical Operator : Logic  AllPortsSameDT=off  OutDataTypeStr=boolean
  Logical Operator1 : Logic  Operator=OR  AllPortsSameDT=off  OutDataTypeStr=boolean
  Product : Product  OutDataTypeStr=single
  Product1 : Product  OutDataTypeStr=single
  Product2 : Product
  Relational Operator : RelationalOperator  Operator=~=  OutDataTypeStr=boolean  RndMeth=Simplest  InputSameDT=off
  Relational Operator1 : RelationalOperator  Operator=~=  OutDataTypeStr=boolean  RndMeth=Simplest  InputSameDT=off
  Sum : Sum  OutDataTypeStr=single  InputSameDT=on  SaturateOnIntegerOverflow=on
  Sum1 : Sum  Inputs=|++  OutDataTypeStr=single
  Switch : Switch  Criteria=u2 ~= 0  SaturateOnIntegerOverflow=off  InputSameDT=off
  Switch1 : Switch  Criteria=u2 ~= 0  SaturateOnIntegerOverflow=off  InputSameDT=off
  Switch2 : Switch  Criteria=u2 ~= 0  SaturateOnIntegerOverflow=off  InputSameDT=off
  Unit Delay : UnitDelay  SampleTime=-1  HasFrameUpgradeWarning=on
  pi_out : Outport  OutDataTypeStr=single  VectorParamsAs1DForOutWhenUnconnected=off
  Uq_out : Outport  Port=2  OutDataTypeStr=single  VectorParamsAs1DForOutWhenUnconnected=off
  wires:
  Product/1 -> Switch2/3, Product1/1  "yp"
  delta_iq/1 -> Product/1  "iq_e"
  iq_p/1 -> Product/2  "iq_e"
  iq_I/1 -> Product1/2  "iq_e"
  Iq_sat/1 -> Switch/3
  Sum1/1 -> Iq_sat1/1
  Product1/1 -> Switch1/3
  Sum/1 -> Iq_sat2/1
  Product2/1 -> Gain/1
  U_dc/1 -> Product2/2
  Gain/1 -> Iq_sat/1
  Switch1/1 -> Sum1/1
  Delay/1 -> Sum1/2
  Switch2/1 -> Sum/1
  Pressure_Cmplt/1 -> Logical Operator/1
  Switch/1 -> Unit Delay/1, pi_out/1
  Unit Delay/1 -> Switch/1
  Constant/1 -> Switch1/1
  Constant1/1 -> Switch2/1
  VCU_Brake_AimPressure/1 -> Relational Operator/1
  Constant2/1 -> Relational Operator/2
  Relational Operator/1 -> Logical Operator/2
  Logical Operator/1 -> Logical Operator1/1, Switch/2
  Iq_sat2/1 -> Product2/1, Uq_out/1
  Constant3/1 -> Relational Operator1/2
  EHB_mode/1 -> Relational Operator1/1
  Logical Operator1/1 -> Switch2/2, Switch1/2
  Relational Operator1/1 -> Logical Operator1/2
  Iq_sat1/1 -> Sum/2, Delay/1

== system EHB_MOTOR/EHB_MOTOR_PRO/Subsystem/SVPWM/Calculate_Phase_Voltages ==
  N : Inport  OutDataTypeStr=uint8
  Ualpha : Inport  Port=2  OutDataTypeStr=single
  Ubeta : Inport  Port=3  OutDataTypeStr=single
  Bus Creator : BusCreator  Inputs=3
  Bus_Voltage : Constant  OutDataTypeStr=single
  Phase_Voltage_Sectors_1_and_4 : Subsystem
  Sector_slect : MultiPortSwitch  Inputs=6  SaturateOnIntegerOverflow=off  InputSameDT=off
  U_Sectors_2_and_5 : Subsystem
  U_Sectors_3_and_6 : Subsystem
  phase_voltages : Outport  VectorParamsAs1DForOutWhenUnconnected=off
  wires:
  Ualpha/1 -> Bus Creator/2  "U_alpha"
  Ubeta/1 -> Bus Creator/3  "U_beta"
  Bus_Voltage/1 -> Bus Creator/1  "Bus_Voltage"
  N/1 -> Sector_slect/1
  Bus Creator/1 -> U_Sectors_3_and_6/1(Bus_Beta), Phase_Voltage_Sectors_1_and_4/1(Bus_Alpha_Beta), U_Sectors_2_and_5/1(Bus_Alpha)
  Sector_slect/1 -> phase_voltages/1
  U_Sectors_3_and_6/1(UVW_Sector_3_and_6) -> Sector_slect/4, Sector_slect/7
  Phase_Voltage_Sectors_1_and_4/1(UVW_Sector_1_and_4) -> Sector_slect/2, Sector_slect/5
  U_Sectors_2_and_5/1(UVW_Sector_2_and_5) -> Sector_slect/6, Sector_slect/3

== system EHB_MOTOR/EHB_MOTOR_PRO/Subsystem/SVPWM/Sector Caculate ==
  note: Phase Advanced Inverse Clarke Transform
  note: Projects the quadrature (beta) component (as opposed to the conventional inverse Clarke transform
      | which projects the alpha component).
  alpha_voltage : Inport
  beta_voltage : Inport  Port=2
  Add : Sum  Inputs=-+
  Add1 : Sum  Inputs=--
  Calculate_Phase_Advanced_Sector : Sum  Inputs=+++  OutDataTypeStr=uint8  AccumDataTypeStr=uint8
  Compare_VA_To_Zero : simulink/Logic and Bit Operations/Compare To Zero  relop=>  OutDataTypeStr=uint8
  Compare_VB_To_Zero : simulink/Logic and Bit Operations/Compare To Zero  relop=>  OutDataTypeStr=uint8
  Compare_VC_To_Zero : simulink/Logic and Bit Operations/Compare To Zero  relop=>  OutDataTypeStr=uint8
  Gain : Gain  Gain=0.5  OutDataTypeStr=Inherit: Same as input
  Gain1 : Gain  Gain=0.866  OutDataTypeStr=Inherit: Same as input
  Sector_Gain_VB : Gain  Gain=2  ParamDataTypeStr=int16  OutDataTypeStr=uint8
  Sector_Gain_VC : Gain  Gain=4  ParamDataTypeStr=int16  OutDataTypeStr=uint8
  Sector_Lookup_Table : LookupNDDirect  NumberOfTableDimensions=1  Table=[2,2,6,1,4,3,5]  TableDataTypeStr=uint8
      settings: AttributesFormatString=-------------------------------\nTable: %<Table>
  sector : Outport  VectorParamsAs1DForOutWhenUnconnected=off
  wires:
  Sector_Gain_VC/1 -> Calculate_Phase_Advanced_Sector/3
  alpha_voltage/1 -> Gain1/1
  Calculate_Phase_Advanced_Sector/1 -> Sector_Lookup_Table/1
  Sector_Lookup_Table/1 -> sector/1
  Compare_VA_To_Zero/1 -> Calculate_Phase_Advanced_Sector/1
  beta_voltage/1 -> Compare_VA_To_Zero/1, Gain/1
  Add1/1 -> Compare_VC_To_Zero/1  "voltage_phase_c"
  Compare_VC_To_Zero/1 -> Sector_Gain_VC/1
  Compare_VB_To_Zero/1 -> Sector_Gain_VB/1
  Sector_Gain_VB/1 -> Calculate_Phase_Advanced_Sector/2
  Gain1/1 -> Add1/2, Add/2
  Gain/1 -> Add1/1, Add/1
  Add/1 -> Compare_VB_To_Zero/1  "voltage_phase_b"

== system EHB_MOTOR/EHB_MOTOR_PRO/Subsystem/Subsystem1/select1_4 ==
  In1 : Inport
  Bus Selector : BusSelector  OutputSignals=Ia_A,Ib_A
  Mux : Mux  Inputs=2
  Out1 : Outport  VectorParamsAs1DForOutWhenUnconnected=off
  wires:
  In1/1 -> Bus Selector/1
  Bus Selector/1 -> Mux/1  "<Ia_A>"
  Bus Selector/2 -> Mux/2  "<Ib_A>"
  Mux/1 -> Out1/1

== system EHB_MOTOR/EHB_MOTOR_PRO/Subsystem/Subsystem1/select2_5 ==
  In1 : Inport
  Add : Sum
  Bus Selector : BusSelector  OutputSignals=Ib_A,Ic_A
  Gain : Gain  Gain=-1
  Mux : Mux  Inputs=2
  Out1 : Outport  VectorParamsAs1DForOutWhenUnconnected=off
  wires:
  In1/1 -> Bus Selector/1
  Bus Selector/1 -> Mux/2, Add/1  "<Ib_A>"
  Bus Selector/2 -> Add/2  "<Ic_A>"
  Add/1 -> Gain/1
  Gain/1 -> Mux/1  "Ia1_6"
  Mux/1 -> Out1/1

== system EHB_MOTOR/EHB_MOTOR_PRO/Subsystem/Subsystem1/select3_6 ==
  In1 : Inport
  Add : Sum
  Bus Selector : BusSelector  OutputSignals=Ia_A,Ic_A
  Gain : Gain  Gain=-1
  Mux : Mux  Inputs=2
  Out1 : Outport  VectorParamsAs1DForOutWhenUnconnected=off
  wires:
  In1/1 -> Bus Selector/1
  Bus Selector/1 -> Mux/1, Add/1  "<Ia_A>"
  Bus Selector/2 -> Add/2  "<Ic_A>"
  Add/1 -> Gain/1
  Gain/1 -> Mux/2  "Ib2_3"
  Mux/1 -> Out1/1

== system EHB_MOTOR/EPB_CTRL/EPB_Diag/EPBCurrentDiag/Subsystem ==
  note: 检测到EPB电机电流超过额定电流
  In1 : Inport
  In2 : Inport  Port=2
  function : TriggerPort  TriggerType=function-call  VariantControl=Variant
  Abs : Abs  SaturateOnIntegerOverflow=off
  Abs1 : Abs  SaturateOnIntegerOverflow=off
  Constant : Constant  Value=0  OutDataTypeStr=uint8
  Data Store Memory1 : DataStoreMemory  DataStoreName=EPBCurrentOverride_C  ReadBeforeWriteMsg=warning  WriteAfterWriteMsg=warning  WriteAfterReadMsg=warning  ShowAdditionalParam=off  OutDataTypeStr=uint16
  Data Store Memory5 : DataStoreMemory  DataStoreName=EPBCurrentMAX_C  ReadBeforeWriteMsg=warning  WriteAfterWriteMsg=warning  WriteAfterReadMsg=warning  ShowAdditionalParam=off  OutDataTypeStr=uint16
  Data Store Read : DataStoreRead  DataStoreName=EPBCurrentOverride_C  DataStoreElements=EPBCurrentOverride_C  IndexOptions=Index vector (dialog)  Indices=1  OutputSizes=1
  Data Store Read2 : DataStoreRead  DataStoreName=EPBCurrentMAX_C  DataStoreElements=EPBCurrentMAX_C  IndexOptions=Index vector (dialog)  Indices=1  OutputSizes=1
  ErrorSignalCount : Stateflow chart  TreatAsAtomicUnit=on
  Logical Operator : Logic  Operator=OR  AllPortsSameDT=off  OutDataTypeStr=boolean
  Relational Operator1 : RelationalOperator  Operator=>  OutDataTypeStr=boolean  RndMeth=Simplest  InputSameDT=off
  Relational Operator2 : RelationalOperator  Operator=>  OutDataTypeStr=boolean  RndMeth=Simplest  InputSameDT=off
  Out1 : Outport  VectorParamsAs1DForOutWhenUnconnected=off
  wires:
  In1/1 -> Abs/1
  Data Store Read2/1 -> Relational Operator2/2, Relational Operator1/2
  ErrorSignalCount/1(EPBCurrentOverride) -> Out1/1
  Data Store Read/1 -> ErrorSignalCount/2(EPBCurrentOverride_C)
  Constant/1 -> ErrorSignalCount/3(Recover)
  Abs/1 -> Relational Operator1/1
  In2/1 -> Abs1/1
  Abs1/1 -> Relational Operator2/1
  Relational Operator1/1 -> Logical Operator/1
  Relational Operator2/1 -> Logical Operator/2
  Logical Operator/1 -> ErrorSignalCount/1(EPBCurrent)
